simulink model "WiperCtrl"  (R2023b)
settings: Solver=FixedStepDiscrete  StartTime=0.0  StopTime=4  FixedStep=5e-5  RelTol=1e-3  EnableMultiTasking=on
values from neighbouring files (symbols this model uses):
  MC_Hardware_Motor_Mechinal_Fric = 0    [ModelParamSet.m]
  MC_Hardware_Motor_Mechinal_Inertia = 1.03e-2    (= 0.0103)    [ModelParamSet.m]
  MC_Hardware_Motor_Mechinal_TF = 8.59e-2    (= 0.0859)    [ModelParamSet.m]
  MC_Hardware_Motor_Rotor_BEMFCoff = 4.294    [ModelParamSet.m]
  MC_Hardware_Motor_Rotor_Pn = 4    [ModelParamSet.m]
  MC_Hardware_Motor_Stator_Ld = 5.6345e-5    (= 5.6345e-05)    [ModelParamSet.m]
  MC_Hardware_Motor_Stator_Lq = 5.6345e-5    (= 5.6345e-05)    [ModelParamSet.m]
  MC_Hardware_Motor_Stator_Rs = 2.86e-2    (= 0.0286)    [ModelParamSet.m]
  MC_Hardware_Power_DC = 13.5    [ModelParamSet.m]
  MC_Hardware_Sample_CurrentNoise = 1e-15    [ModelParamSet.m]
  MC_Hardware_Sample_Rs = 1e-3    (= 0.001)    [ModelParamSet.m]
  MC_Hardware_Sample_VbusNoise = 1e-15    [ModelParamSet.m]
  MC_Sim_BaseStep = 5e-8    (= 5e-08)    [ModelParamSet.m]
  MC_Sim_HighFrequenceStep = 5e-5    (= 5e-05)    [ModelParamSet.m]
  MC_SVPWM_DutyMax = 0.98    [ModelParamSet.m]
  MC_SVPWM_DutyMin = 0.02    [ModelParamSet.m]
libraries: simulink x12, spsVoltageMeasurementLib x2, spsDCVoltageSourceLib x1, spsGroundLib x1, spsPermanentMagnetSynchronousMachineLib x1, spsSeriesRLCBranchLib x1, spsThreePhaseVIMeasurementLib x1, spsUniversalBridgeLib x1, spspowerguiLib x1
(part 2 of 2)

== system WiperCtrl/HighFrequency/svpwm/invClarkeTransform/invClarkeTransform ==
  Valpha : Inport
  Vbeta : Inport  Port=2
  Add : Sum
  Gain : Gain  Gain=-1/2
  Gain1 : Gain  Gain=sqrt(3)/2
  Subtract : Sum  Inputs=+-
  Va : Outport
  Vb : Outport  Port=2
  Vc : Outport  Port=3
  wires:
  Valpha/1 -> Gain/1, Va/1  "Va"
  Vbeta/1 -> Gain1/1
  Gain/1 -> Subtract/1, Add/1
  Gain1/1 -> Subtract/2, Add/2
  Add/1 -> Vb/1  "Vb"
  Subtract/1 -> Vc/1  "Vc"

== system WiperCtrl/Hardware_Math/CurrentSample/CurrentSample(OneRS) /CurrentSample2/CurrentSample2Down ==
  Current : Inport
  Trigger : TriggerPort  TriggerType=falling  VariantControl=(inherit)  InitialTriggerSignalState=zero
  ADCOffset : Constant  Value=0  SampleTime=-1
  ADCQuality : Gain  Gain=1024/5
  Add : Sum
  CSAGain : Gain  Gain=50
  CurrentSample2 : Outport
  wires:
  ADCQuality/1 -> CurrentSample2/1
  ADCOffset/1 -> Add/1
  Add/1 -> ADCQuality/1
  CSAGain/1 -> Add/2
  Current/1 -> CSAGain/1

== system WiperCtrl/Hardware_Math/CurrentSample/CurrentSample(OneRS) /CurrentSample2/CurrentSample2Up ==
  Current : Inport
  Trigger : TriggerPort  VariantControl=(inherit)  InitialTriggerSignalState=zero
  ADCOffset : Constant
  ADCQuality : Gain
  Add : Sum
  CSAGain : Gain
  CurrentSample2 : Outport
  wires:
  ADCQuality/1 -> CurrentSample2/1
  ADCOffset/1 -> Add/1
  CSAGain/1 -> Add/2
  Add/1 -> ADCQuality/1
  Current/1 -> CSAGain/1

== system WiperCtrl/HighFrequency/svpwm/getDutyandSample/dutyExchange/gateHtoPhase ==
  SectorN : Inport
  DutyLH : Inport  Port=2
  DutyMH : Inport  Port=3
  DutySH : Inport  Port=4
  Constant : Constant
  Multiport Switch : MultiPortSwitch  DataPortOrder=Zero-based contiguous  Inputs=8  zeroidx=on  SaturateOnIntegerOverflow=off  InputSameDT=off
  Multiport Switch1 : MultiPortSwitch  DataPortOrder=Zero-based contiguous  Inputs=8  zeroidx=on  SaturateOnIntegerOverflow=off  InputSameDT=off
  Multiport Switch2 : MultiPortSwitch  DataPortOrder=Zero-based contiguous  Inputs=8  zeroidx=on  SaturateOnIntegerOverflow=off  InputSameDT=off
  Mux : Mux  Inputs=3
  GateH : Outport
  wires:
  SectorN/1 -> Multiport Switch2/1, Multiport Switch1/1, Multiport Switch/1
  Constant/1 -> Multiport Switch2/9, Multiport Switch2/2, Multiport Switch1/9, Multiport Switch1/2, Multiport Switch/9, Multiport Switch/2
  Multiport Switch/1 -> Mux/1
  Multiport Switch1/1 -> Mux/2
  Multiport Switch2/1 -> Mux/3
  Mux/1 -> GateH/1
  DutyLH/1 -> Multiport Switch2/8, Multiport Switch2/6, Multiport Switch1/7, Multiport Switch1/3, Multiport Switch/5, Multiport Switch/4
  DutyMH/1 -> Multiport Switch2/7, Multiport Switch2/4, Multiport Switch1/6, Multiport Switch1/5, Multiport Switch/8, Multiport Switch/3
  DutySH/1 -> Multiport Switch2/5, Multiport Switch2/3, Multiport Switch1/8, Multiport Switch1/4, Multiport Switch/7, Multiport Switch/6

== system WiperCtrl/HighFrequency/svpwm/getDutyandSample/dutyExchange/gateLtoPhase ==
  SectorN : Inport
  DutyLH : Inport  Port=2
  DutyMH : Inport  Port=3
  DutySH : Inport  Port=4
  Constant : Constant
  Multiport Switch : MultiPortSwitch  DataPortOrder=Zero-based contiguous  Inputs=8  zeroidx=on  SaturateOnIntegerOverflow=off  InputSameDT=off
  Multiport Switch1 : MultiPortSwitch  DataPortOrder=Zero-based contiguous  Inputs=8  zeroidx=on  SaturateOnIntegerOverflow=off  InputSameDT=off
  Multiport Switch2 : MultiPortSwitch  DataPortOrder=Zero-based contiguous  Inputs=8  zeroidx=on  SaturateOnIntegerOverflow=off  InputSameDT=off
  Mux : Mux  Inputs=3
  GateL : Outport
  wires:
  DutySH/1 -> Multiport Switch/6, Multiport Switch/7, Multiport Switch1/4, Multiport Switch1/8, Multiport Switch2/3, Multiport Switch2/5
  DutyMH/1 -> Multiport Switch/3, Multiport Switch/8, Multiport Switch1/5, Multiport Switch1/6, Multiport Switch2/4, Multiport Switch2/7
  DutyLH/1 -> Multiport Switch/4, Multiport Switch/5, Multiport Switch1/3, Multiport Switch1/7, Multiport Switch2/6, Multiport Switch2/8
  Mux/1 -> GateL/1
  Multiport Switch2/1 -> Mux/3
  Multiport Switch1/1 -> Mux/2
  Multiport Switch/1 -> Mux/1
  Constant/1 -> Multiport Switch/2, Multiport Switch/9, Multiport Switch1/2, Multiport Switch1/9, Multiport Switch2/2, Multiport Switch2/9
  SectorN/1 -> Multiport Switch/1, Multiport Switch1/1, Multiport Switch2/1

== system WiperCtrl/HighFrequency/svpwm/getDutyandSample/getV/getVmax ==
  Va : Inport
  Vb : Inport  Port=2
  Vc : Inport  Port=3
  Relational Operator : RelationalOperator  OutDataTypeStr=boolean  RndMeth=Simplest  InputSameDT=off
  Relational Operator1 : RelationalOperator  OutDataTypeStr=boolean  RndMeth=Simplest  InputSameDT=off
  Switch : Switch  Criteria=u2 > Threshold  SaturateOnIntegerOverflow=off  InputSameDT=off
  Switch1 : Switch  Criteria=u2 > Threshold  SaturateOnIntegerOverflow=off  InputSameDT=off
  Vmax : Outport
  wires:
  Va/1 -> Relational Operator/1, Switch/1
  Vb/1 -> Relational Operator/2, Switch/3
  Relational Operator/1 -> Switch/2
  Switch/1 -> Relational Operator1/1, Switch1/1
  Vc/1 -> Relational Operator1/2, Switch1/3
  Relational Operator1/1 -> Switch1/2
  Switch1/1 -> Vmax/1  "Vmax"

== system WiperCtrl/HighFrequency/svpwm/getDutyandSample/getV/getVmin ==
  Va : Inport
  Vb : Inport  Port=2
  Vc : Inport  Port=3
  Relational Operator1 : RelationalOperator  Operator=<=  OutDataTypeStr=boolean  RndMeth=Simplest  InputSameDT=off
  Relational Operator2 : RelationalOperator  Operator=<=  OutDataTypeStr=boolean  RndMeth=Simplest  InputSameDT=off
  Switch : Switch  Criteria=u2 > Threshold  SaturateOnIntegerOverflow=off  InputSameDT=off
  Switch1 : Switch  Criteria=u2 > Threshold  SaturateOnIntegerOverflow=off  InputSameDT=off
  Vmin : Outport
  wires:
  Switch1/1 -> Vmin/1  "Vmin"
  Relational Operator2/1 -> Switch1/2
  Vc/1 -> Relational Operator2/2, Switch1/3
  Switch/1 -> Relational Operator2/1, Switch1/1
  Relational Operator1/1 -> Switch/2
  Vb/1 -> Relational Operator1/2, Switch/3
  Va/1 -> Relational Operator1/1, Switch/1
